simulink model "Schloss_Box_final"  (R2017b)
settings: Solver=FixedStepAuto  StartTime=0.0  StopTime=10.0  RelTol=1e-3
PreLoadFcn:
  | waijung.modelPreload; % Required for working with Waijung Blockset. Do not remove.
undefined symbols (not defined in the file): Blocking, HSEOSC, Link, LQFP100, Non, ST, STM32F407VG
libraries: stm32f4_canbus_lib x4, simulink x4, stm32f4_io_lib x4, hdlsllib x2, stm32f4_device_config_lib x1
CloseFcn:
  | waijung.modelClose; % Required for working with Waijung Blockset. Do not remove.
settings Model: Creator=labuser  LastModifiedBy=labuser
settings OptimizationCC: DefaultParameterBehavior=Inlined  PassReuseOutputArgsAs=Individual arguments
settings DebuggingCC: ParameterTunabilityLossMsg=error
settings HardwareCC: ProdBitPerPointer=32  ProdBitPerSizeT=32  ProdBitPerPtrDiffT=32  ProdLargestAtomicFloat=None  ProdIntDivRoundTo=Undefined  ProdWordSize=32  ProdHWDeviceType=ARM Compatible->Cortex - M4  TargetEndianess=LittleEndian  TargetHWDeviceType=ARM Compatible->Cortex - M4
settings SFSimCC: MATLABDynamicMemAlloc=off
settings RTWCC: SystemTargetFile=stm32f4.tlc  GenerateMakefile=off  TemplateMakefile=ert_default_tmf  Description=STM32F4 Target  GenerateReport=on  IncludeHyperlinkInReport=on  LaunchReport=on  GenerateTraceInfo=on  GenerateTraceReport=on  GenerateTraceReportSl=on  GenerateTraceReportSf=on  GenerateTraceReportEml=on
settings CodeAppCC: ForceParamTrailComments=on  IgnoreCustomStorageClasses=off  OperatorAnnotations=on  SimulinkDataObjDesc=on  SFDataObjDesc=on  InsertBlockDesc=on
settings STFCustomTargetCC: TargetLangStandard=C99 (ISO)  MultiwordLength=256  ModelReferenceCompliant=off  CombineOutputUpdateFcns=on  ERTCustomFileBanners=on  SupportContinuousTime=off  SupportNonInlinedSFcns=off  RemoveResetFunc=on  MATLABClassNameForMDSCustomization=Simulink.SoftwareTarget.ERTCustomization  GRTInterface=off  SystemTargetFile=stm32f4.tlc
settings ERTTargetCC: TargetLangStandard=C99 (ISO)  ModelReferenceCompliant=off  ParMdlRefBuildCompliant=off  CompOptLevelCompliant=off  ConcurrentExecutionCompliant=off  ModelStepFunctionPrototypeControlCompliant=off  CPPClassGenCompliant=off  UseToolchainInfoCompliant=off  InlinedParameterPlacement=NonHierarchical  ERTSrcFileBannerTemplate=stm32f4_code_template.cgt  ERTHdrFileBannerTemplate=stm32f4_code_template.cgt  ERTDataSrcFileTemplate=stm32f4_code_template.cgt  ERTDataHdrFileTemplate=stm32f4_code_template.cgt  ERTCustomFileTemplate=stm32f4_file_process.tlc

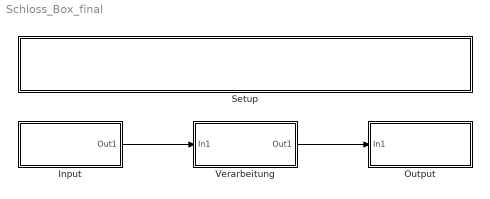
== system Schloss_Box_final ==
  Input : Subsystem
  Output : Subsystem
  Setup : Subsystem
  Verarbeitung : Subsystem
  wires:
  Input/1(Out1) -> Verarbeitung/1(In1)
  Verarbeitung/1(Out1) -> Output/1(In1)

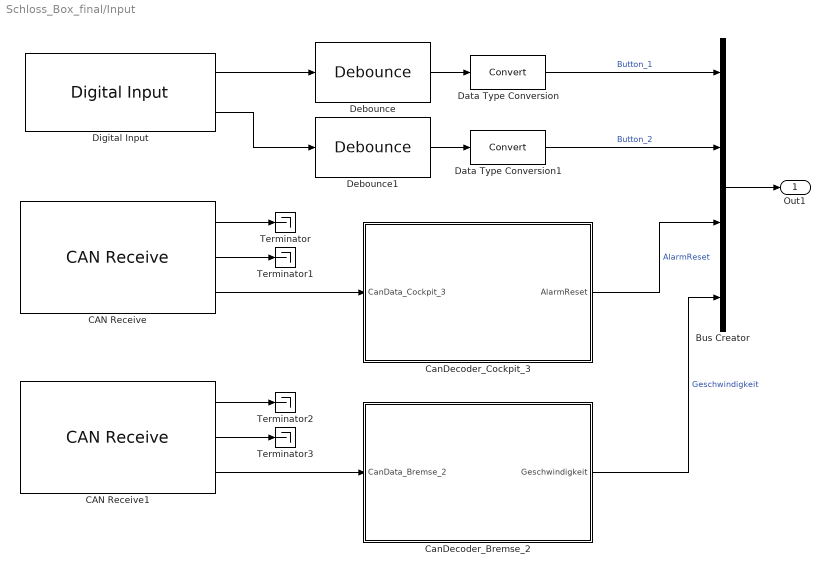
== system Schloss_Box_final/Input ==
  Bus Creator : BusCreator  Inputs=4
  CAN Receive : stm32f4_canbus_lib/CAN Receive  conf=Rx  canmodule=1  idtype=Standard  filtertype=Specific  id=18  idmask=00000000  enableisr=off  usedlc=off  datatype=single  data0type=uint8  data1type=Not used  data2type=Not used  data3type=Not used  data4type=Not used  data5type=Not used  data6type=Not used  data7type=Not used  buffersize=8  sampletime=-1  sampletimestr=-1  blockid=InputCANReceive  inputarray=[]  inputlabelarray={}  outputarray=[ 5, 7, 3]  outputlabelarray={ 'Msg Pending','ID', 'D0 (uint8)' }  compat=0  confstr="[\"Standard\",\"Specific\",\"18\",\"0\",\"off\",\"uint8\",\"Not used\",\"Not used\",\"Not used\",\"Not used\",\"Not used\",\"Not used\",\"Not used\",\"8\",\"240\",\"0\",\"FFE0\",\"4\"]"
      settings: SourceProductName=Waijung Blockset
  CAN Receive1 : stm32f4_canbus_lib/CAN Receive  conf=Rx  canmodule=1  idtype=Standard  filtertype=Specific  id=12  idmask=00000000  enableisr=off  usedlc=off  datatype=single  data0type=uint8  data1type=Not used  data2type=Not used  data3type=Not used  data4type=Not used  data5type=Not used  data6type=Not used  data7type=Not used  buffersize=8  sampletime=-1  sampletimestr=-1  blockid=InputCANReceive1  inputarray=[]  inputlabelarray={}  outputarray=[ 5, 7, 3]  outputlabelarray={ 'Msg Pending','ID', 'D0 (uint8)' }  compat=0  confstr="[\"Standard\",\"Specific\",\"12\",\"0\",\"off\",\"uint8\",\"Not used\",\"Not used\",\"Not used\",\"Not used\",\"Not used\",\"Not used\",\"Not used\",\"8\",\"180\",\"0\",\"FFE0\",\"4\"]"
      settings: SourceProductName=Waijung Blockset
  CanDecoder_Bremse_2 : Subsystem
  CanDecoder_Cockpit_3 : Subsystem
  Data Type Conversion : DataTypeConversion
  Data Type Conversion1 : DataTypeConversion
  Debounce : stm32f4_io_lib/Debounce  mode=Single Pulse  prescale=4  debounce=4
      settings: SourceProductName=Waijung Blockset
  Debounce1 : stm32f4_io_lib/Debounce  mode=Single Pulse  prescale=4  debounce=4
      settings: SourceProductName=Waijung Blockset
  Digital Input : stm32f4_io_lib/Digital Input  port=C  speed=100  porttype=None  porttypestr=NOPULL  use_pin0=on  use_pin1=on  use_pin2=off  use_pin3=off  use_pin4=off  use_pin5=off  use_pin6=off  use_pin7=off  use_pin8=off  use_pin9=off  use_pin10=off  use_pin11=off  use_pin12=off  use_pin13=off  use_pin14=off  use_pin15=off  pinstr=GPIO_Pin_0 | GPIO_Pin_1  usedpinarray="[1  1  0  0  0  0  0  0  0  0  0  0  0  0  0  0]"  bitbandingstr=|  sampletime=-1  sampletimestr=-1  blockid=InputDigitalInput  enablecustomportlabel=off  glabalinit=off  cinputportlabel=In1, In2  coutputportlabel=Out1, Out2
      | #define InputDigitalInput_C0 Peripheral_BB(GPIOC->IDR, 0)  /* Output pin */
      | #define InputDigitalInput_C1 Peripheral_BB(GPIOC->IDR, 1)  /* Output pin */
      settings: SourceProductName=Waijung Blockset
  Terminator{,1..3} (4 alike) : Terminator
  Out1 : Outport
  wires:
  Bus Creator/1 -> Out1/1
  CAN Receive/2 -> Terminator1/1
  CanDecoder_Bremse_2/1(Geschwindigkeit) -> Bus Creator/4  "Geschwindigkeit"
  CAN Receive1/3 -> CanDecoder_Bremse_2/1(CanData_Bremse_2)
  Data Type Conversion/1 -> Bus Creator/1  "Button_1"
  CAN Receive/3 -> CanDecoder_Cockpit_3/1(CanData_Cockpit_3)
  CAN Receive1/2 -> Terminator3/1
  Debounce1/1 -> Data Type Conversion1/1
  Data Type Conversion1/1 -> Bus Creator/2  "Button_2"
  Digital Input/2 -> Debounce1/1
  CanDecoder_Cockpit_3/1(AlarmReset) -> Bus Creator/3  "AlarmReset"
  Debounce/1 -> Data Type Conversion/1
  CAN Receive1/1 -> Terminator2/1
  Digital Input/1 -> Debounce/1
  CAN Receive/1 -> Terminator/1

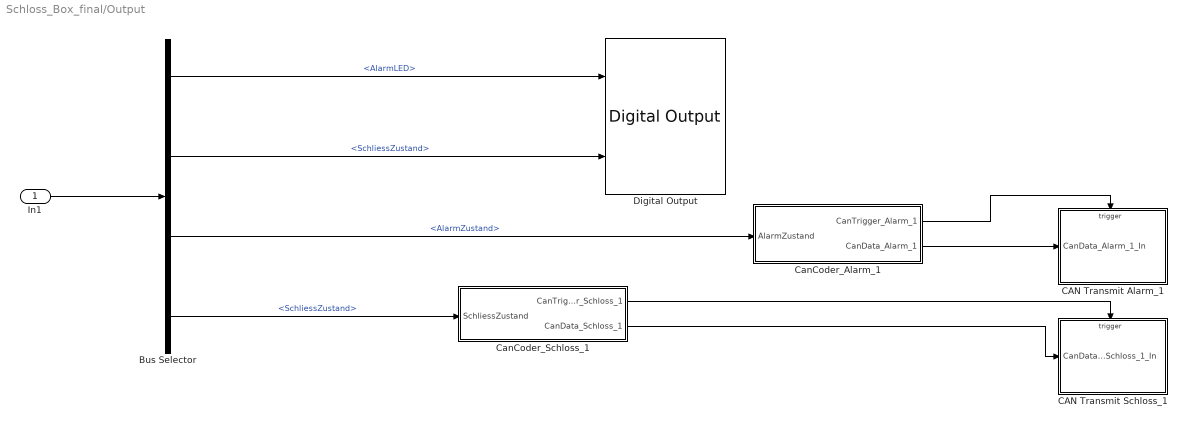
== system Schloss_Box_final/Output ==
  In1 : Inport
  Bus Selector : BusSelector  OutputSignals=AlarmLED,SchliessZustand,AlarmZustand,SchliessZustand
  CAN Transmit Alarm_1 : Subsystem  TreatAsAtomicUnit=on
  CAN Transmit Schloss_1 : Subsystem  TreatAsAtomicUnit=on
  CanCoder_Alarm_1 : Subsystem
  CanCoder_Schloss_1 : Subsystem
  Digital Output : stm32f4_io_lib/Digital Output  use_bitband=on  port=C  speed=100  porttype=Push Pull  porttypestr=PP  use_pin0=off  use_pin1=off  use_pin2=on  use_pin3=on  use_pin4=off  use_pin5=off  use_pin6=off  use_pin7=off  use_pin8=off  use_pin9=off  use_pin10=off  use_pin11=off  use_pin12=off  use_pin13=off  use_pin14=off  use_pin15=off  pinstr=GPIO_Pin_2 | GPIO_Pin_3  usedpinarray="[0  0  1  1  0  0  0  0  0  0  0  0  0  0  0  0]"  bitbandingstr=|  sampletime=-1  sampletimestr=-1  blockid=OutputDigitalOutput  enablecustomportlabel=off  globalinit=off  cinputportlabel=In1, In2  coutputportlabel=0
      | #define OutputDigitalOutput_C2 Peripheral_BB(GPIOC->ODR, 2)  /* Output pin */
      | #define OutputDigitalOutput_C3 Peripheral_BB(GPIOC->ODR, 3)  /* Output pin */
      settings: SourceProductName=Waijung Blockset
  wires:
  In1/1 -> Bus Selector/1
  CanCoder_Schloss_1/2(CanData_Schloss_1) -> CAN Transmit Schloss_1/1(CanData_Schloss_1_In)
  CanCoder_Alarm_1/2(CanData_Alarm_1) -> CAN Transmit Alarm_1/1(CanData_Alarm_1_In)
  CanCoder_Alarm_1/1(CanTrigger_Alarm_1) -> CAN Transmit Alarm_1/Trigger
  Bus Selector/2 -> Digital Output/2  "<SchliessZustand>"
  Bus Selector/4 -> CanCoder_Schloss_1/1(SchliessZustand)  "<SchliessZustand>"
  CanCoder_Schloss_1/1(CanTrigger_Schloss_1) -> CAN Transmit Schloss_1/Trigger
  Bus Selector/1 -> Digital Output/1  "<AlarmLED>"
  Bus Selector/3 -> CanCoder_Alarm_1/1(AlarmZustand)  "<AlarmZustand>"

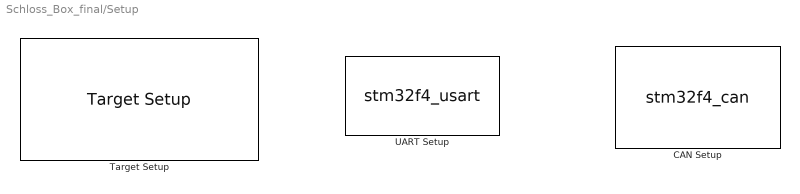
== system Schloss_Box_final/Setup ==
  CAN Setup : S-Function  FunctionName=stm32f4_can  Parameters=conf,canmodule,0,inputarray,outputarray,'','',confstr,sampletime,sampletimestr,blockid  SFunctionDeploymentMode=off  EnableBusSupport=off  mask(stm32f4_can){conf=Setup, canmodule=1, advance=off, bitrate_select=125000, sjw=1tq, bs1=14tq, bs2=6tq, timingconf=Prescaler, brp=16, bitrate=125000, tq=3.8095e-07, autoretransmission=Disable, remaptxpin=D1, remaprxpin=D0, sampletime=-1, sampletimestr=-1, blockid=SetupCANSetup, inputarray=[], inputlabelarray={}, outputarray=[], outputlabelarray={}, compat=0, confstr=["125000","16","D","1","D","0","1tq","14tq","6tq","ENABLE"], presc=16, txportstr=D, txpinstr=1, rxportstr=D, rxpinstr=0, lastmodule=1}
      mask prompts: conf "Configuration"; canmodule "CAN Module"; advance "Advance configuration"; bitrate_select "Baud rate (bps)"; sjw "Resync Jump Width (SJW)"; bs1 "Bit segment 1 (BS1) + PROP_SEG"; bs2 "Bit segment 2 (BS2)"; timingconf "Adjust"; brp "Baud rate prescaler (BRP)"; bitrate "Baud rate (bps)"; tq "Time Quantum (Second), tq"; autoretransmission "Auto Re-transmission"; remaptxpin "CAN Tx pin"; remaprxpin "CAN Rx pin"; sampletime "Sample time (sec)"; sampletimestr "Compiled sample time (sec) in string"; inputarray "Input port"; inputlabelarray "Input port label"; outputarray "Output port"; outputlabelarray "Output port label"; compat "Compatibility (Reserved for future use)"; confstr "Configuration String"; presc "Prescale"; txportstr "Tx port string"; txpinstr "Tx pin string"; rxportstr "Rx port string"; rxpinstr "Rx pin string"; lastmodule "Last module selected"
      mask help:
      | This block setups CAN Module.
      |
      | Auto Re-transmission,
      |  - Enable: The CAN hardware will automatically retransmit the message until it has been
      | successfully transmitted according to the CAN standard.
      |  - Disable: A message will be transmitted only once, independently of the transmission result
      | (successful, error or arbitration lost).
      mask init:
      | stm32f4_can_callback('init');
      mask Help: web(fullfile(waijungdocroot,'stm32f4_can_setup.htm'), '-browser')
      mask TypeOptions conf: Setup
      mask TypeOptions canmodule: 1 | 2
      mask Callback canmodule: stm32f4_can_callback('canmodule');
      mask Callback advance: stm32f4_can_callback('advance');
      mask TypeOptions bitrate_select: 125000 | 250000 | 500000 | 1000000
      mask Callback bitrate_select: stm32f4_can_callback('bitrate_select');
      mask TypeOptions sjw: 1tq | 2tq | 3tq | 4tq
      mask TypeOptions bs1: 1tq | 2tq | 3tq | 4tq | 5tq | 6tq | 7tq | 8tq | 9tq | 10tq | 11tq | 12tq | 13tq | 14tq | 15tq | 16tq
      mask Callback bs1: stm32f4_can_callback('timingconf');
      mask TypeOptions bs2: 1tq | 2tq | 3tq | 4tq | 5tq | 6tq | 7tq | 8tq
      mask Callback bs2: stm32f4_can_callback('timingconf');
      mask TypeOptions timingconf: Prescaler | Baudrate
      mask Callback timingconf: stm32f4_can_callback('timingconf');
      mask Callback brp: stm32f4_can_callback('timingconf');
      mask Callback bitrate: stm32f4_can_callback('timingconf');
      mask TypeOptions autoretransmission: Enable | Disable
      mask TypeOptions remaptxpin: Not used | A12 | B9 | D1
      mask Callback remaptxpin: stm32f4_can_callback('remaptxpin');
      mask TypeOptions remaprxpin: Not used | A11 | B8 | D0
      mask Callback remaprxpin: stm32f4_can_callback('remaprxpin');
      mask Callback sampletime: stm32f4_can_callback('sampletime');
      mask Callback sampletimestr: stm32f4_can_callback('sampletimestr');
      mask Callback blockid: stm32f4_can_callback('blockid');
      mask Display: text(0.5, 0.5, 'CAN1_Setup\nSpeed (bps): 125000\nTx/Rx pin: D1/D0','ver','middle','hor','center');
  Target Setup : stm32f4_device_config_lib/Target Setup  Priority=100  compiler=GNU ARM  previous_compiler=GNU ARM  mcu=STM32F407VG (LQFP100)  mcustr=STM32F407VG  clockconfig=HSEOSC-8MHz  system_stm32f4xx_c_path=C:\Users\labuser\Desktop\waijung17_03a\targets\stm32f4_target\stm32f4\utils\system_stm32f4xx_default\STM32F40_41xxx\hseosc8mhz  showmemoryconfiguration=off  stacksize=0x2000  heapsize=0x2000  enableautocompiledownload=on  fullchiperase=off  programmerinterface=ST-Link  editctrlstr=on  compilercontrolstr=$(patsubst %, -I%, .) -mcpu=cortex-m4 -mthumb -mthumb-interwork -mfloat-abi=hard -mfpu=fpv4-sp-d16 -ffast-math -Wall -Wextra -Ofast  assemblercontrolstr=$(patsubst %, -I%, .) -mcpu=cortex-m4 -mthumb -mthumb-interwork -mfloat-abi=hard -mfpu=fpv4-sp-d16 -ffast-math -Wall -Wextra -Ofast -Wa,-amhls=$(<:.s=.lst) -D__STACK_SIZE=$(STACK_SIZE) -D__HEAP_SIZE=$(HEAP_SIZE)  linkercontrolstr=-T$(LD_SCRIPT) -g -Wl,-Map=$(MAP),--cref,--no-warn-mismatch -mcpu=cortex-m4 -mthumb -mthumb-interwork -mfloat-abi=hard -mfpu=fpv4-sp-d16 -specs=nosys.specs  runafterdownload=on  execprofile=None  profileruart=3  profilerbaud=500000  profilertxpin=D8  profilerinitstr=0.01,168000000,1680000,500000,0  manualsetsampletime=off  sampletime=0.01  blockid=SetupTargetSetup  systickreloadvalue=1680000  hseval=8000000  lastprofileruart=3  hclk=168000000  flashorigin=0x8000000  flashlength=1024k  ramorigin=0x20000000  ramlength=128k  useextram=off
      settings: SourceProductName=Waijung Blockset
  UART Setup : S-Function  Priority=1  FunctionName=stm32f4_usart  Parameters=configuration,uartmodule,transfer,baudrate,inputtype,outputtype,confstr,binheaderarray,binterminatorarray,asciiheader,asciiterminator,bindatalength,packetmode,varname,sampletime,sampletimestr,blockid  SFunctionDeploymentMode=off  EnableBusSupport=off  mask(stm32f4_usart){configuration=Setup, uartmodule=2, baudrate=115200, databits=8, parity=No, stopbit=1, remaptxpin=A2, remaprxpin=A3, flowcontrol=None, remapctspin=Not used, remaprtspin=Not used, advanceoptions=off, rxbuffersize=512, txbuffersize=512, transfer=Blocking, packetmode=Ascii, binheader='7E 7E', binterminator='03 03', porttype_double=1, porttype_single=0, porttype_int8=1, porttype_uint8=0, porttype_int16=0, porttype_uint16=0, porttype_int32=0, porttype_uint32=0, asciiformat='%d,%f', rx_asciiterminator=CRLF (0x0D 0x0A - "\r\n"), tx_asciiterminator=CR (0x0D - "\r"), storagename=<empty>, varname=, inputtype=[0], outputtype=[0], binheaderarray=[0], binterminatorarray=[0], bindatalength=0, asciiheader='', asciiterminator=[0], sampletime=-1, sampletimestr=-1, blockid=SetupUARTSetup, confstr=[ "dummy", "1", "A", "2", "1", "A", "3", "0", "*", "*", "0", "*", "*", "1", "4", "6", "1", "4", "5", "512", "512", "1", "2", "115200", "8", "No", "1", "None", "USART2"], lastmodule=2}
      mask prompts: uartmodule "UART Module"; baudrate "Baud rate (bps)"; databits "Data bits"; stopbit "Stop bit"; remaptxpin "Tx Pin"; remaprxpin "Rx Pin"; flowcontrol "Hardware flow control"; remapctspin "HW Flow control, CTS Pin"; remaprtspin "HW Flow control, RTS Pin"; advanceoptions "Advance options"; rxbuffersize "Rx buffer size (bytes)"; txbuffersize "Tx buffer size (bytes)"; packetmode "Packet mode"; binheader "Binary header (example: '7E 7E')"; binterminator "Binary terminator (example: '03 03')"; porttype_double "Number of data port, type DOUBLE"; porttype_single "Number of data port, type SINGLE"; porttype_int8 "Number of data port, type INT8"; porttype_uint8 "Number of data port, type UINT8"; porttype_int16 "Number of data port, type INT16"; porttype_uint16 "Number of data port, type UINT16"; porttype_int32 "Number of data port, type INT32"; porttype_uint32 "Number of data port, type UINT32"; asciiformat "Ascii format"; rx_asciiterminator "End of packet"; tx_asciiterminator "End of packet"; storagename "Buffer"; varname "Var name"; inputtype "Input data type"; outputtype "Output data type"; binheaderarray "Binary header"; binterminatorarray "Binary terminator"; bindatalength "Binary data length"; asciiheader "Ascii header (printf format)"; asciiterminator "Ascii terminator"; sampletime "Sample time (sec)"; sampletimestr "Compiled sample time (sec) in string"; confstr "Configuration string"; lastmodule "Last module selected"
      mask help:
      | Default STM32F4DISCOVERY + aMG F4 Connect 2 + aMG USB Converter N2 settings use
      |
      | USART3, Tx D8, Rx D9 and USB Serial Converter A.
      mask init:
      | stm32f4_usart_callback('init');
      mask Help: web(fullfile(waijungdocroot,'stm32f4_usart_setup.htm'), '-browser')
      mask TypeOptions configuration: Setup | Tx | Rx
      mask Callback configuration: stm32f4_usart_callback('configuration');
      mask TypeOptions uartmodule: 1 | 2 | 3 | 4 | 5 | 6
      mask Callback uartmodule: stm32f4_usart_callback('uartmodule');
      mask Callback baudrate: stm32f4_usart_callback('baudrate');
      mask TypeOptions databits: 8
      mask TypeOptions parity: No | Odd | Even
      mask TypeOptions stopbit: 0.5 | 1 | 1.5 | 2
      mask TypeOptions remaptxpin: Not used | A2 | D5
      mask TypeOptions remaprxpin: Not used | A3 | D6
      mask TypeOptions flowcontrol: None | RTS | CTS | RTS/CTS
      mask Callback flowcontrol: stm32f4_usart_callback('flowcontrol');
      mask TypeOptions remapctspin: Not used | A0 | D3
      mask TypeOptions remaprtspin: Not used | A1 | D4
      mask Callback advanceoptions: stm32f4_usart_callback('advanceoptions');
      mask TypeOptions rxbuffersize: 16 | 32 | 64 | 128 | 256 | 512 | 1024 | 2048
      mask TypeOptions txbuffersize: 16 | 32 | 64 | 128 | 256 | 512 | 1024 | 2048
      mask TypeOptions transfer: Blocking | Non-Blocking
      mask Callback transfer: stm32f4_usart_callback('transfer');
      mask TypeOptions packetmode: Ascii | Binary | String Buffer
      mask Callback packetmode: stm32f4_usart_callback('packetmode');
      mask Callback binheader: stm32f4_usart_callback('binheader');
      mask Callback binterminator: stm32f4_usart_callback('binterminator');
      mask Callback porttype_double: stm32f4_usart_callback('porttype');
      mask Callback porttype_single: stm32f4_usart_callback('porttype');
      mask Callback porttype_int8: stm32f4_usart_callback('porttype');
      mask Callback porttype_uint8: stm32f4_usart_callback('porttype');
      mask Callback porttype_int16: stm32f4_usart_callback('porttype');
      mask Callback porttype_uint16: stm32f4_usart_callback('porttype');
      mask Callback porttype_int32: stm32f4_usart_callback('porttype');
      mask Callback porttype_uint32: stm32f4_usart_callback('porttype');
      mask Callback asciiformat: stm32f4_usart_callback('asciiformat');
      mask TypeOptions rx_asciiterminator: CR (0x0D - "\r") | LF (0x0A - "\n") | CRLF (0x0D 0x0A - "\r\n")
      mask Callback rx_asciiterminator: stm32f4_usart_callback('rx_asciiterminator');
      mask TypeOptions tx_asciiterminator: CR (0x0D - "\r") | LF (0x0A - "\n") | CRLF (0x0D 0x0A - "\r\n") | None
      mask Callback tx_asciiterminator: stm32f4_usart_callback('tx_asciiterminator');
      mask TypeOptions storagename: <empty>
      mask Callback storagename: stm32f4_usart_callback('storagename');
      mask Callback varname: stm32f4_usart_callback('varname');
      mask Callback sampletime: stm32f4_usart_callback('sampletime');
      mask Callback sampletimestr: stm32f4_usart_callback('sampletimestr');
      mask Callback blockid: stm32f4_usart_callback('blockid');
      mask Display: text(0.5, 0.5, 'Module: USART2_Setup\nBaud (Bps): 115200\nDMA Buffer: 512/512\nTx/Rx Pin: A2/A3','ver','middle','hor','center');

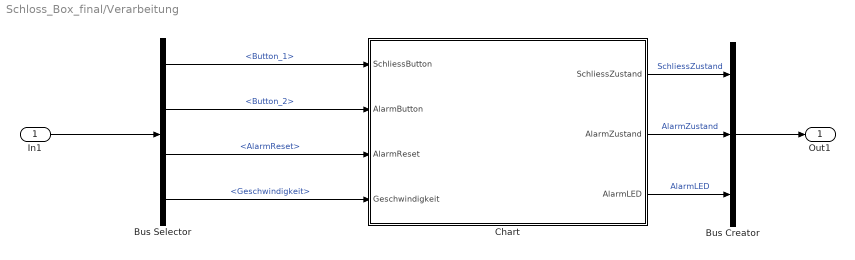
== system Schloss_Box_final/Verarbeitung ==
  In1 : Inport
  Bus Creator : BusCreator  Inputs=3
  Bus Selector : BusSelector  OutputSignals=Button_1,Button_2,AlarmReset,Geschwindigkeit
  Chart : Stateflow chart  TreatAsAtomicUnit=on
  Out1 : Outport
  wires:
  Bus Creator/1 -> Out1/1
  In1/1 -> Bus Selector/1
  Bus Selector/2 -> Chart/2(AlarmButton)  "<Button_2>"
  Bus Selector/1 -> Chart/1(SchliessButton)  "<Button_1>"
  Bus Selector/3 -> Chart/3(AlarmReset)  "<AlarmReset>"
  Bus Selector/4 -> Chart/4(Geschwindigkeit)  "<Geschwindigkeit>"
  Chart/1(SchliessZustand) -> Bus Creator/1  "SchliessZustand"
  Chart/2(AlarmZustand) -> Bus Creator/2  "AlarmZustand"
  Chart/3(AlarmLED) -> Bus Creator/3  "AlarmLED"

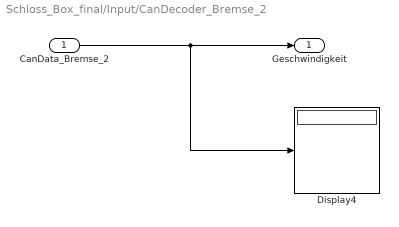
== system Schloss_Box_final/Input/CanDecoder_Bremse_2 ==
  CanData_Bremse_2 : Inport
  Display4 : Display
  Geschwindigkeit : Outport
  wires:
  CanData_Bremse_2/1 -> Display4/1, Geschwindigkeit/1

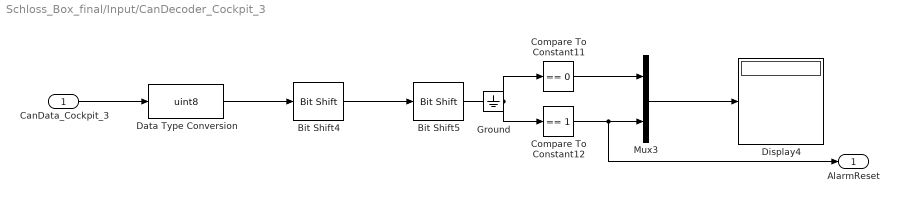
== system Schloss_Box_final/Input/CanDecoder_Cockpit_3 ==
  CanData_Cockpit_3 : Inport
  Bit Shift4 : hdlsllib/Logic and Bit Operations/Bit Shift  mode=Shift Left Logical  N=7
      settings: SourceProductName=HDL Coder  SourceProductBaseCode=HD
  Bit Shift5 : hdlsllib/Logic and Bit Operations/Bit Shift  mode=Shift Right Logical  N=7
      settings: SourceProductName=HDL Coder  SourceProductBaseCode=HD
  Compare To Constant11 : simulink/Logic and Bit Operations/Compare To Constant  relop===  const=0  OutDataTypeStr=boolean
  Compare To Constant12 : simulink/Logic and Bit Operations/Compare To Constant  relop===  const=1  OutDataTypeStr=boolean
  Data Type Conversion : DataTypeConversion  OutDataTypeStr=uint8
  Display4 : Display
  Ground : Ground
  Mux3 : Mux  Inputs=2
  AlarmReset : Outport
  wires:
  Compare To Constant11/1 -> Mux3/1
  Bit Shift4/1 -> Bit Shift5/1
  Bit Shift5/1 -> Compare To Constant11/1, Compare To Constant12/1
  CanData_Cockpit_3/1 -> Data Type Conversion/1
  Compare To Constant12/1 -> AlarmReset/1, Mux3/2
  Data Type Conversion/1 -> Bit Shift4/1
  Mux3/1 -> Display4/1

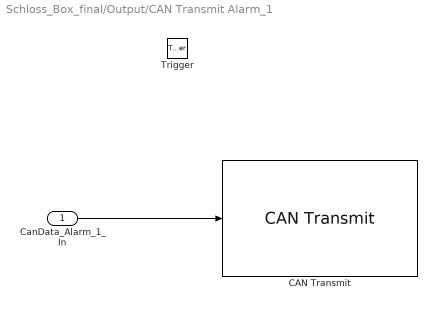
== system Schloss_Box_final/Output/CAN Transmit Alarm_1 ==
  CanData_Alarm_1_In : Inport
  Trigger : TriggerPort  VariantControl=Variant
  CAN Transmit : stm32f4_canbus_lib/CAN Transmit  conf=Tx  canmodule=1  transfer=Non-Blocking  timeout=0.005  idtype=Standard  specificid=on  id=24  specificdlc=on  dlc=1  enablestatus=off  datatype=single  data0type=uint8  data1type=Not used  data2type=Not used  data3type=Not used  data4type=Not used  data5type=Not used  data6type=Not used  data7type=Not used  inputarray=[ 3]  inputlabelarray={ 'D0 (uint8)' }  outputarray=[]  outputlabelarray={}  sampletime=-1  sampletimestr=-1  blockid=OutputCANTransmitAlarm_1CANTransmit  compat=0  confstr="[\"Non-Blocking\",\"0.005\",\"Standard\",\"on\",\"24\",\"on\",\"1\",\"off\",\"uint8\",\"Not used\",\"Not used\",\"Not used\",\"Not used\",\"Not used\",\"Not used\",\"Not used\"]"
      settings: SourceProductName=Waijung Blockset
  wires:
  CanData_Alarm_1_In/1 -> CAN Transmit/1

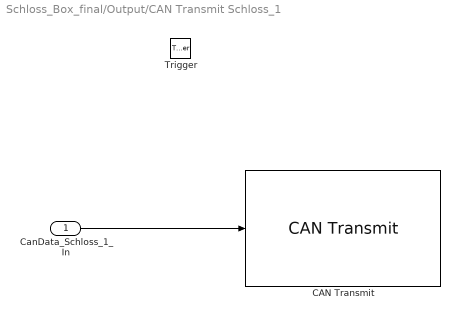
== system Schloss_Box_final/Output/CAN Transmit Schloss_1 ==
  CanData_Schloss_1_In : Inport
  Trigger : TriggerPort  VariantControl=Variant
  CAN Transmit : stm32f4_canbus_lib/CAN Transmit  conf=Tx  canmodule=1  transfer=Non-Blocking  timeout=0.005  idtype=Standard  specificid=on  id=25  specificdlc=on  dlc=1  enablestatus=off  datatype=single  data0type=uint8  data1type=Not used  data2type=Not used  data3type=Not used  data4type=Not used  data5type=Not used  data6type=Not used  data7type=Not used  inputarray=[ 3]  inputlabelarray={ 'D0 (uint8)' }  outputarray=[]  outputlabelarray={}  sampletime=-1  sampletimestr=-1  blockid=OutputCANTransmitSchloss_1CANTransmit  compat=0  confstr="[\"Non-Blocking\",\"0.005\",\"Standard\",\"on\",\"25\",\"on\",\"1\",\"off\",\"uint8\",\"Not used\",\"Not used\",\"Not used\",\"Not used\",\"Not used\",\"Not used\",\"Not used\"]"
      settings: SourceProductName=Waijung Blockset
  wires:
  CanData_Schloss_1_In/1 -> CAN Transmit/1

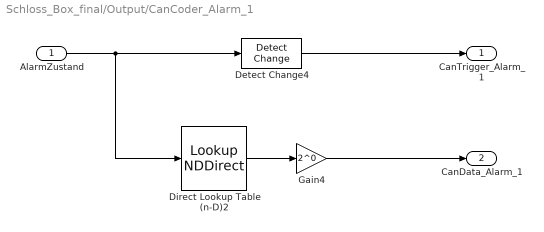
== system Schloss_Box_final/Output/CanCoder_Alarm_1 ==
  AlarmZustand : Inport
  Detect Change4 : simulink/Logic and Bit Operations/Detect Change  vinit=0  OutDataTypeStr=boolean
  Direct Lookup Table (n-D)2 : LookupNDDirect  NumberOfTableDimensions=1  Table=[0; 1]
  Gain4 : Gain  Gain=2^0  OutDataTypeStr=uint8
  CanTrigger_Alarm_1 : Outport
  CanData_Alarm_1 : Outport  Port=2
  wires:
  Direct Lookup Table (n-D)2/1 -> Gain4/1
  Gain4/1 -> CanData_Alarm_1/1
  AlarmZustand/1 -> Detect Change4/1, Direct Lookup Table (n-D)2/1
  Detect Change4/1 -> CanTrigger_Alarm_1/1

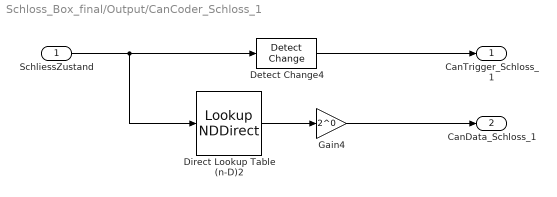
== system Schloss_Box_final/Output/CanCoder_Schloss_1 ==
  SchliessZustand : Inport
  Detect Change4 : simulink/Logic and Bit Operations/Detect Change  vinit=0  OutDataTypeStr=boolean
  Direct Lookup Table (n-D)2 : LookupNDDirect  NumberOfTableDimensions=1  Table=[0; 1]
  Gain4 : Gain  Gain=2^0  OutDataTypeStr=uint8
  CanTrigger_Schloss_1 : Outport
  CanData_Schloss_1 : Outport  Port=2
  wires:
  Gain4/1 -> CanData_Schloss_1/1
  Detect Change4/1 -> CanTrigger_Schloss_1/1
  Direct Lookup Table (n-D)2/1 -> Gain4/1
  SchliessZustand/1 -> Detect Change4/1, Direct Lookup Table (n-D)2/1

== stateflow chart Schloss_Box_final/Verarbeitung/Chart ==
  state Schliessanlage [parallel]
    settings: executionOrder=1
    state Geschlossen
      entry: SchliessZustand=1
    state OFFEN
      entry: SchliessZustand=0
    (default) -> Geschlossen
    Geschlossen -> OFFEN : [SchliessButton==1]
    OFFEN -> Geschlossen : [SchliessButton==1]
  state Alarmanlage [parallel]
    settings: executionOrder=2
    state OFF
      entry: AlarmLED=false;
    state ON
      state TRIGGER_ON
        entry: AlarmZustand=1
      state TRIGGER_OFF
        entry:AlarmZustand=0
        state LED
          entry:
          AlarmLED=(~AlarmLED);
        (default) -> LED
        LED -> LED : after(1,sec)
      (default) -> TRIGGER_OFF
      TRIGGER_OFF -> TRIGGER_ON [order 1] : [AlarmButton==1]
      TRIGGER_ON -> TRIGGER_OFF : [SchliessZustand==0&&AlarmReset==1]
    (default) -> OFF
    OFF -> ON : [SchliessZustand==1 && Geschwindigkeit==0]
    TRIGGER_OFF -> OFF [order 2] : [SchliessZustand==0]
  data: SchliessButton input; AlarmButton input; SchliessZustand output; AlarmZustand output; AlarmReset input; Geschwindigkeit input; Trigger_Zustand constant boolean; AlarmLED output boolean
